simulink model "AirplaneSimModel_AutomaticTrajectory"  (R2018b)
settings: Solver=ode4  StartTime=0.0  StopTime=30  FixedStep=0.001  RelTol=1e-3
undefined symbols (not defined in the file): aileron_left, aileron_right, airplane, alt_ground, atmosphere, B_aileron_p_14ms, B_elevator_q_14ms, B_rudder_r_14ms, elevator, envir, g, htp_trim, inital_vel_vec, K_atti, K_lateral, K_vertical, rudder, throttle, traj, wind
libraries: actuators_lib x11, unit_conversions_lib x6, axes_transformation_lib x2, quatAttitudeController_lib x2, conventional_airplane_single_engine_lib x1, atmosphere_lib x1, sensors_lib x1, simulink x1, flightgear_visualization_lib x1
(part 2 of 2)

== matlab function AirplaneSimModel_AutomaticTrajectory/QuaternionAttitudeController/DCM 2 q_bg continuous4/MATLAB Function3 ==
  data: M_bg input; q_bg output; last_q input
function q_bg  = dcm2QuatCont( M_bg, last_q )

% dcm2Quat computes the quaternion (q_bg) from the direction cosine matrix
% (DCM) so that there are no discontinuities.
%   The quaternion is used to represent the attitude of the body
%   relative to the earth. It can be computed from the DCM. However, there
%   exist two solutions with reversed signs. This function avoids steps
%   which can be important for controllers.
% 
% Literature:
%   [1] Wu, J. (2018). Optimal Continuous Unit Quaternions from Rotation
%       Matrices. Journal of Guidance, Control and Dynamics.
% 
% Inputs:
%   M_bg            direction cosine matrix (with 3x3 elements) from NED
%                   frame (g) to body frame (b).
% 
% Outputs:
%   q_bg            quaternion vector with 4 elements and euclean norm of 1
% 
% See also: dcm2Quat
% 

% Disclaimer:
%   SPDX-License-Identifier: GPL-3.0-only
% 
%   Copyright (C) 2020-2022 Yannic Beyer
%   Copyright (C) 2022 TU Braunschweig, Institute of Flight Guidance
% *************************************************************************

% get quaternions (with discontinuities)

%q_bg = dcm2Quat( M_bg );
q_bg = rotm2quat(M_bg)';

% remove discontinuities
q_bg = sign(q_bg' * last_q) * q_bg;


end

== matlab function AirplaneSimModel_AutomaticTrajectory/AoA Compensation Backup/AOA Calc1/MATLAB Function ==
  data: V input; alpha output; C_A input; S input; az input; m input; rho input
function alpha = calculateAoA(V, C_A, S, az, m, rho)

alpha = az * m / max((rho/2 * V^2 * C_A * S), eps);

end

== matlab function AirplaneSimModel_AutomaticTrajectory/Measurements1/MATLAB Function5 ==
  data: u input; y output
function y = fcn(u)

y = norm(u);

== matlab function AirplaneSimModel_AutomaticTrajectory/QuaternionAttitudeController/MATLAB Function1 ==
  data: I input; Q_b output; omega_Kb input; dot_omega_Kb_cmd input
function Q_b = fcn(I,omega_Kb,dot_omega_Kb_cmd)

Q_b = I * dot_omega_Kb_cmd + cross( omega_Kb, I * omega_Kb );

end
